simulink model "questB_LQR_model"  (R2018a)
settings: Solver=VariableStepAuto  StartTime=0.0  StopTime=14  RelTol=1e-3
values from neighbouring files (symbols this model uses):
  A = [0 1 0 0; 20.6 0 0 0; 0 0 0 1; -.5 0 0 0]    [InvertedPendulum.m]
  B = [0; -1; 0; .5]    [InvertedPendulum.m]
  C = [1 0 0 0; 0 0 1 0]    [InvertedPendulum.m]
  x0 = [-.2; -.06; .01; .3]    [InvertedPendulum.m]
undefined symbols (not defined in the file or in its folder): K_lqr
settings Model: Creator=patsa  LastModifiedBy=patsa

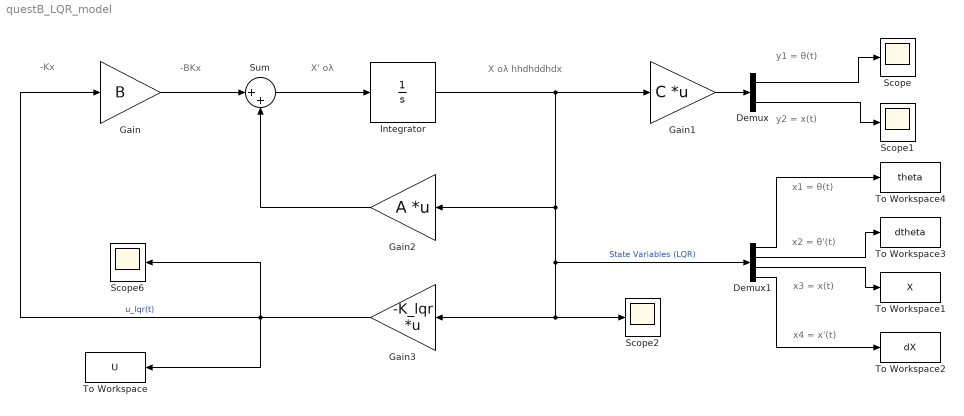
== system questB_LQR_model ==
  note: x1 = θ(t)
  note: -Kx
  note: y2 = x(t)
  note: -BKx
  note: X ολ
      |
      | hhdhddhdx
  note: y1 = θ(t)
  note: x2 = θ'(t)
  note: x3 = x(t)
  note: X' ολ
  note: x4 = x'(t)
  Demux : Demux  Outputs=2
  Demux1 : Demux
  Gain : Gain  Gain=B
  Gain1 : Gain  Gain=C  Multiplication=Matrix(K*u)
  Gain2 : Gain  Gain=A  Multiplication=Matrix(K*u)
  Gain3 : Gain  Gain=-K_lqr  Multiplication=Matrix(K*u)
  Integrator : Integrator  InitialCondition=x0
  Scope{,1..2,6} (4 alike) : Scope
  Sum : Sum  Inputs=|++
  To Workspace : ToWorkspace  VariableName=U  SaveFormat=Timeseries  SampleTime=1
  To Workspace1 : ToWorkspace  VariableName=X  SaveFormat=Timeseries  SampleTime=1
  To Workspace2 : ToWorkspace  VariableName=dX  SaveFormat=Timeseries  SampleTime=1
  To Workspace3 : ToWorkspace  VariableName=dtheta  SaveFormat=Timeseries  SampleTime=1
  To Workspace4 : ToWorkspace  VariableName=theta  SaveFormat=Timeseries  SampleTime=1
  wires:
  Demux/2 -> Scope1/1
  Gain2/1 -> Sum/2
  Gain/1 -> Sum/1
  Integrator/1 -> Gain1/1, Scope2/1, Gain3/1, Demux1/1, Gain2/1  "State Variables (LQR)"
  Gain3/1 -> To Workspace/1, Gain/1, Scope6/1  "u_lqr(t)"
  Gain1/1 -> Demux/1
  Demux1/2 -> To Workspace3/1
  Demux1/1 -> To Workspace4/1
  Demux1/3 -> To Workspace1/1
  Sum/1 -> Integrator/1
  Demux/1 -> Scope/1
  Demux1/4 -> To Workspace2/1
